simulink model "SINGLE_PHASE_INVERTER_PR_CONTROLLER"  (R2023a)
settings: Solver=ode45  StartTime=0.0  StopTime=0.05  MaxStep=1e-7  MinStep=1e-8  RelTol=1e-3
libraries: spsIGBTDiodeLib x4, spsSeriesRLCBranchLib x4, spsCurrentMeasurementLib x2, spsDCVoltageSourceLib x1, simulink x1, spsVoltageMeasurementLib x1, sps_lib x1
settings Model: Creator=sudib  LastModifiedBy=sudib

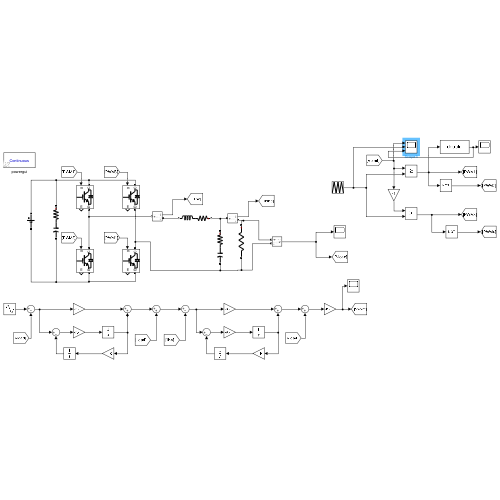
[thumbnail: Simulink's stored preview of the top-level diagram]
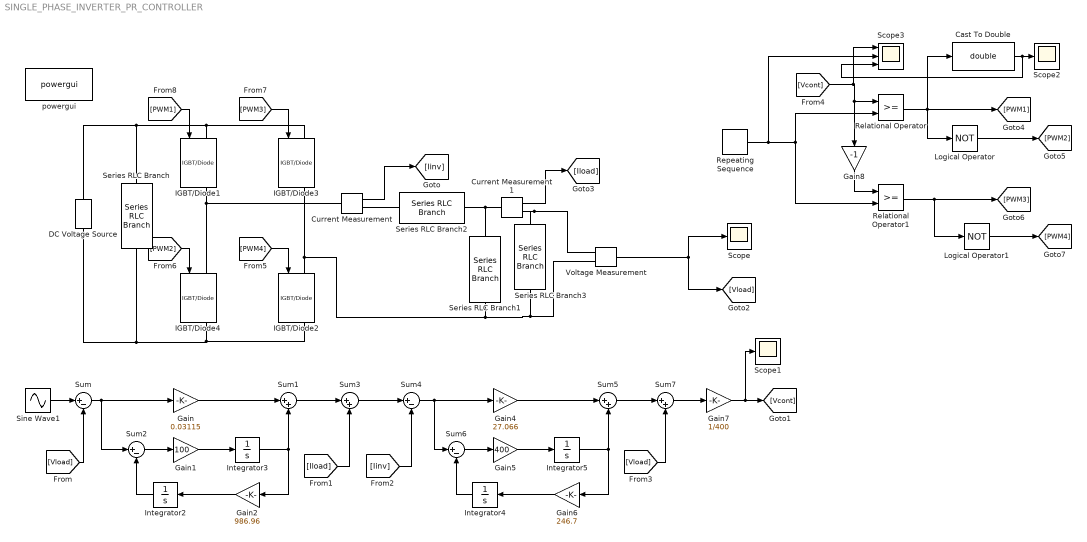
== system SINGLE_PHASE_INVERTER_PR_CONTROLLER ==
  Cast To Double : DataTypeConversion  OutDataTypeStr=double  SaturateOnIntegerOverflow=off  RndMeth=Floor
  Current Measurement : spsCurrentMeasurementLib/Current Measurement  PhasorSimulation=off  OutputType=Complex  PSBequivalent=0
  Current Measurement1 : spsCurrentMeasurementLib/Current Measurement  PhasorSimulation=off  OutputType=Complex  PSBequivalent=0
  DC Voltage Source : spsDCVoltageSourceLib/DC Voltage Source  Amplitude=400  Measurements=None
  Gain : Gain  Gain=0.03115
  Gain1 : Gain  Gain=100
  Gain2 : Gain  Gain=986.96
  Gain4 : Gain  Gain=27.066
  Gain5 : Gain  Gain=400
  Gain6 : Gain  Gain=246.7
  Gain7 : Gain  Gain=1/400
  Gain8 : Gain  Gain=-1
  IGBT/Diode{1..4} (4 alike) : spsIGBTDiodeLib/IGBT//Diode  Ron=1e-3  Rs=1e5  Cs=inf  Measurements=on
  Integrator{2..5} (4 alike) : Integrator
  Logical Operator : Logic  Operator=NOT  AllPortsSameDT=off  OutDataTypeStr=boolean
  Logical Operator1 : Logic  Operator=NOT  AllPortsSameDT=off  OutDataTypeStr=boolean
  Relational Operator : RelationalOperator  OutDataTypeStr=boolean  RndMeth=Simplest  InputSameDT=off
  Relational Operator1 : RelationalOperator  OutDataTypeStr=boolean  RndMeth=Simplest  InputSameDT=off
  Repeating Sequence : simulink/Sources/Repeating Sequence  rep_seq_t=[0 0.00005 0.0001]  rep_seq_y=[-1 1 -1]
  Scope : Scope
  Scope1 : Scope
  Scope2 : Scope
  Scope3 : Scope  NumInputPorts=3
  Series RLC Branch : spsSeriesRLCBranchLib/Series RLC Branch  LConnTagsString=__new0  RConnTagsString=__new0  BranchType=RC  Resistance=0.001  Inductance=1e-3  SetiL0=off  InitialCurrent=0  Capacitance=500e-6  Setx0=off  InitialVoltage=0  Measurements=None
  Series RLC Branch1 : spsSeriesRLCBranchLib/Series RLC Branch  LConnTagsString=__new0  RConnTagsString=__new0  BranchType=RC  Resistance=0.0042  Inductance=1e-3  SetiL0=off  InitialCurrent=0  Capacitance=6.23e-6  Setx0=off  InitialVoltage=0  Measurements=None
  Series RLC Branch2 : spsSeriesRLCBranchLib/Series RLC Branch  LConnTagsString=__new0  RConnTagsString=__new0  BranchType=RL  Resistance=0.001  Inductance=4.06e-3  SetiL0=off  InitialCurrent=0  Capacitance=1e-6  Setx0=off  InitialVoltage=0  Measurements=None
  Series RLC Branch3 : spsSeriesRLCBranchLib/Series RLC Branch  LConnTagsString=__new0  RConnTagsString=__new0  BranchType=R  Resistance=55  Inductance=1e-3  SetiL0=off  InitialCurrent=0  Capacitance=6.23e-6  Setx0=off  InitialVoltage=0  Measurements=None
  Sine Wave1 : Sin  Amplitude=400  Frequency=314.14  SampleTime=0
  Sum{,2,4,6} (4 alike) : Sum  Inputs=|+-
  Sum{1,3,5,7} (4 alike) : Sum  Inputs=|++
  Voltage Measurement : spsVoltageMeasurementLib/Voltage Measurement  PhasorSimulation=off  OutputType=Complex  PSBequivalent=0
  powergui : sps_lib/powergui  Priority=1  SimulationMode=Continuous  SampleTime=50e-6  frequency=60  Iterations=50  frequencyindice=0  Pbase=100e6  ErrMax=1e-4  UnitsV=kV  UnitsW=MW  buscounter=0  FunctionMessages=off  echomessages=off  EnableUseOfTLC=off  CurrentSourceSwitches=off  DisableSnubberDevices=off  DisableRonSwitches=off  DisableVfSwitches=off  DisplayEquations=off  AutomaticDiscreteSolvers=off  SolverType=Tustin/Backward Euler (TBE)  Interpol=off  ExternalGateDelay=off  methode=off  Ts=100  x0status=blocks  SPID=on  SwTol=0  HookPort=off  NonlinearTolerance=1e-4  nMaxIteration=100  ContinueOnMaxIteration=off  RestoreLinks=warning  ResistiveCurrentMeasurement=off  Frange=[0:2:500]  Ylog=off  Xlog=on  ShowGrid=off  save=off  variable=ZData  structure=0  ZoomFFT=off  StartTime=0.0  cycles=1  DisplayStyle=1  fundamental=60  FreqAxis=off  MaxFrequency=1000  frequencyindicesteady=1  RmsSteady=1  display=off
  wires:
  Current Measurement/1 -> [Iinv]
  Voltage Measurement/1 -> [Vload], Scope/1
  Sum/1 -> Sum2/1, Gain/1
  Gain/1 -> Sum1/1
  Gain1/1 -> Integrator3/1
  Integrator3/1 -> Gain2/1, Sum1/2
  Gain2/1 -> Integrator2/1
  Sum2/1 -> Gain1/1
  Integrator2/1 -> Sum2/2
  [Vload] -> Sum/2
  Sine Wave1/1 -> Sum/1
  Sum6/1 -> Gain5/1
  Integrator5/1 -> Gain6/1, Sum5/2
  Integrator4/1 -> Sum6/2
  Gain4/1 -> Sum5/1
  Gain6/1 -> Integrator4/1
  Gain5/1 -> Integrator5/1
  [Iload] -> Sum3/2
  Sum1/1 -> Sum3/1
  Sum3/1 -> Sum4/1
  [Iinv] -> Sum4/2
  Sum4/1 -> Sum6/1, Gain4/1
  Sum5/1 -> Sum7/1
  [Vload] -> Sum7/2
  Sum7/1 -> Gain7/1
  Gain7/1 -> Scope1/1, [Vcont]
  Current Measurement1/1 -> [Iload]
  [Vcont] -> Scope3/1, Gain8/1, Relational Operator/1
  Gain8/1 -> Relational Operator1/1
  Repeating Sequence/1 -> Scope3/2, Relational Operator1/2, Relational Operator/2
  Relational Operator1/1 -> Logical Operator1/1, [PWM3]
  Relational Operator/1 -> Cast To Double/1, [PWM1], Logical Operator/1
  Logical Operator1/1 -> [PWM4]
  Logical Operator/1 -> [PWM2]
  [PWM4] -> IGBT/Diode2/1
  [PWM3] -> IGBT/Diode3/1
  [PWM1] -> IGBT/Diode1/1
  [PWM2] -> IGBT/Diode4/1
  Cast To Double/1 -> Scope3/3, Scope2/1
  connections:
  DC Voltage Source/RConn1 -- IGBT/Diode3/LConn1 -- IGBT/Diode1/LConn1 -- Series RLC Branch/LConn1
  IGBT/Diode4/RConn1 -- IGBT/Diode2/RConn1 -- DC Voltage Source/LConn1 -- Series RLC Branch/RConn1
  IGBT/Diode1/RConn1 -- Current Measurement/LConn1 -- IGBT/Diode4/LConn1
  IGBT/Diode3/RConn1 -- Series RLC Branch3/RConn1 -- Voltage Measurement/LConn2 -- Series RLC Branch1/RConn1 -- IGBT/Diode2/LConn1
  Series RLC Branch2/RConn1 -- Current Measurement/RConn1
  Series RLC Branch3/LConn1 -- Current Measurement1/RConn1 -- Voltage Measurement/LConn1
  Series RLC Branch2/LConn1 -- Current Measurement1/LConn1 -- Series RLC Branch1/LConn1
